simulink library "GainLibrary"  (R2022b)
settings: Solver=VariableStepAuto  StartTime=0.0  StopTime=10.0  RelTol=1e-3
libraries: AudioStats x1
settings Model: Creator=kl13806  LastModifiedBy=kl13806
settings SolverCC: AlgebraicLoopSolver=TrustRegion
settings DebuggingCC: UnconnectedInputMsg=warning  UnconnectedOutputMsg=warning  UnconnectedLineMsg=warning  SFMachineParentedDataDiag=warning  ArithmeticOperatorsInVariantConditions=warning
settings ModelReferenceCC: EnableRefExpFcnMdlSchedulingChecks=on
settings SFSimCC: SimUseLocalCustomCode=off  CustomCodeUndefinedFunction=UseInterfaceOnly
settings RTWCC: RTWUseLocalCustomCode=off  DLArmComputeVersion=19.05
settings CodeAppCC: StateflowObjectComments=on

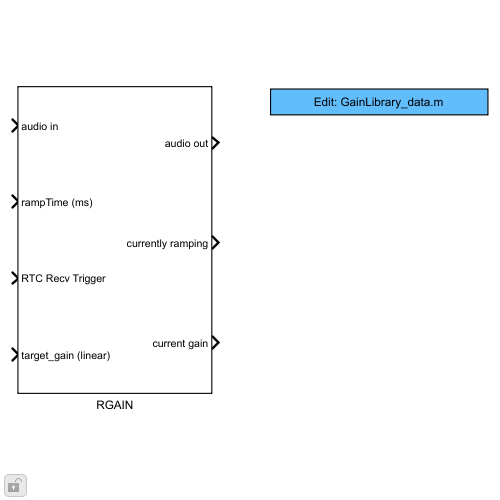
[thumbnail: Simulink's stored preview of the top-level diagram]
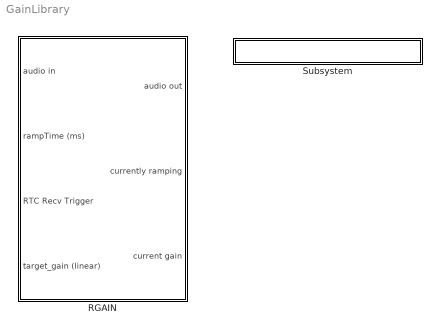
== system GainLibrary ==
  RGAIN : Subsystem  mask(Bose RGAIN){initial_linear_gain=1}
      mask prompts: initial_linear_gain "Initial gain (linear)"
      mask help: The RGAIN block applies a single target gain to all input audio channels.
      mask init:
      | MASK_CONTROL_INIT.frameCount = 0;
      | MASK_CONTROL_INIT.rampCoeff = 1;
      | MASK_CONTROL_INIT.targetGain = initial_linear_gain;
      | MASK_CONTROL_INIT.currentGain = initial_linear_gain;
  Subsystem : Subsystem  mask{filename=GainLibrary_data.m}
      settings: OpenFcn=edit(get(gcbh,'filename'));
      mask Display: disp(['Edit: ' get(gcbh,'filename')]);

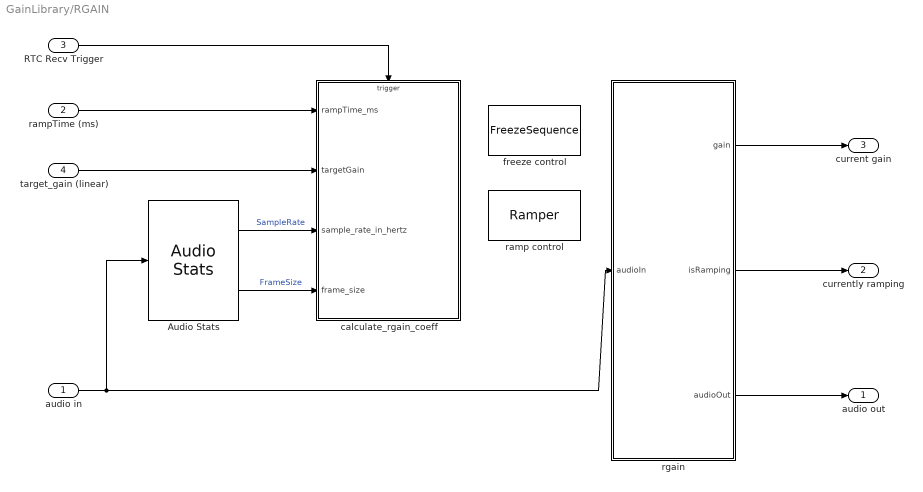
== system GainLibrary/RGAIN ==
  audio in : Inport
  rampTime (ms) : Inport  Port=2
  RTC Recv Trigger : Inport  Port=3
  target_gain (linear) : Inport  Port=4
  Audio Stats : AudioStats/Audio Stats  macroNameRoot=AUDIO  doSampleRate=on  typeSampleRate=Inherit: auto  validateSampleRate=off  valueSampleRate=44100  macroSampleRate=off  doCallRate=off  typeCallRate=Inherit: auto  validateCallRate=off  valueCallRate=[]  macroCallRate=off  doFrameSize=on  typeFrameSize=Inherit: auto  validateFrameSize=off  valueFrameSize=32  macroFrameSize=off  doChannelCount=off  typeChannelCount=Inherit: auto  validateChannelCount=off  valueChannelCount=2  macroChannelCount=off  doTaskRateFactor=off  typeTaskRateFactor=Inherit: auto  validateTaskRateFactor=off  valueTaskRateFactor=[]  macroTaskRateFactor=off  macroTaskID=off
  calculate_rgain_coeff : MATLAB Function  TreatAsAtomicUnit=on
  freeze control : DataStoreMemory  DataStoreName=FreezeSequence  InitialValue=[0,0]  ShowAdditionalParam=off  OutDataTypeStr=uint32
  ramp control : DataStoreMemory  DataStoreName=Ramper  InitialValue=MASK_CONTROL_INIT  ShowAdditionalParam=off  OutDataTypeStr=Bus: rgain_bus
  rgain : MATLAB Function  TreatAsAtomicUnit=on
  audio out : Outport  VectorParamsAs1DForOutWhenUnconnected=off
  currently ramping : Outport  Port=2  VectorParamsAs1DForOutWhenUnconnected=off
  current gain : Outport  Port=3  VectorParamsAs1DForOutWhenUnconnected=off
  wires:
  Audio Stats/1 -> calculate_rgain_coeff/3(sample_rate_in_hertz)  "SampleRate"
  rgain/2(isRamping) -> currently ramping/1
  RTC Recv Trigger/1 -> calculate_rgain_coeff/Trigger
  target_gain (linear)/1 -> calculate_rgain_coeff/2(targetGain)
  rampTime (ms)/1 -> calculate_rgain_coeff/1(rampTime_ms)
  rgain/1(gain) -> current gain/1
  rgain/3(audioOut) -> audio out/1
  audio in/1 -> Audio Stats/1, rgain/1(audioIn)
  Audio Stats/2 -> calculate_rgain_coeff/4(frame_size)  "FrameSize"

== system GainLibrary/Subsystem ==

== matlab function GainLibrary/RGAIN/calculate_rgain_coeff ==
  data: rampTime_ms input; targetGain input; sample_rate_in_hertz input; frame_size input; Ramper data_store_memory; rgain_SILENT_GAIN parameter; FreezeSequence data_store_memory
  events: trigger input FUNCTION_CALL_EVENT
function calculate_rgain_coeff(...
     rampTime_ms, targetGain, sample_rate_in_hertz, frame_size, rgain_SILENT_GAIN)
%#codegen

global Ramper;
global FreezeSequence;


% Step 1: FREEZE the gain ramper so that we can perform calculations based
% on the current gain value. Also, record the control sequence number used
% to specify this soon-to-be-calculated target state.
FreezeSequence(1) = uint32(1); % freeze the gain
FreezeSequence(2) = uint32(1234); % and remember the control sequence (TBD - more changes coming here)

currentGain = Ramper.currentGain;

% Step 2: Nudge the gain values a bit if they are sitting at zero.
% When this control set goes live, ensure that the current gain will move.
% If current gain is zero, replace with a value very close to zero. What we
% really want is a value which is on the edge of perception - not too small
% or large. If the value is too small, we'll waste some of our ramp time
% in perceived silence. If the value is too large, the audio will lurch
% into perceptability at the start of the ramp.
currentGain = max(currentGain, rgain_SILENT_GAIN);

% Step 3: QUANTIZE the desired ramp time to our FrameSize. Also retrieve 
% the whole number of frames required to best match requested ramp time.
% Ensure that at least one frame is used. The frame size will therefore
% determine the steepest ramp (i.e. within one frame you can go anywhere).
quantum_ms = 1000 * frame_size / sample_rate_in_hertz;
numFrames = single(rampTime_ms) / quantum_ms;
numFrames = max (1, round(numFrames));
quantized_rampTime_ms = numFrames * quantum_ms;

%   In order to have the desired ramp time, the slope must vary dependent on the gain difference
%   between target and current value.
%   Ramper's coefficient is therefore calculated as follows:
%                log(TargetGain/CurrentGain)
%   RampCoef = ------------------------------
%                   Fs*(RampTime_ms/1000)
%
factor = log( max(targetGain, rgain_SILENT_GAIN) / currentGain );
RampCoef = exp(factor / (sample_rate_in_hertz * quantized_rampTime_ms / 1000));

% Output asynchronous control signals
Ramper.frameCount   = int32( numFrames );
Ramper.rampCoeff    = single(RampCoef);
Ramper.targetGain   = targetGain;
Ramper.currentGain  = currentGain;

% Release the full rate processing to perform the ramp
FreezeSequence(1) = FreezeSequence(1) - uint32(1);

== matlab function GainLibrary/RGAIN/rgain ==
  data: gain output; isRamping output; audioIn input; audioOut output; Ramper data_store_memory; FreezeSequence data_store_memory
function [gain, isRamping, audioOut]  = rgain(audioIn)
%#codegen

global Ramper;
global FreezeSequence;

% set the size of the output buffer
audioOut = coder.nullcopy(audioIn);

% figure out the frame size
[frame_size, channel_count] = size(audioIn);

% Unpack the control info
frameCount = Ramper.frameCount;
rampCoeff = Ramper.rampCoeff;
targetGain = Ramper.targetGain;
gain = Ramper.currentGain;

% Determine whether gain is ramping or not
% Assume the ramp is frozen
isRamping = false;
k = single(1);

if (FreezeSequence(1) == false)
    if (frameCount == 0)
        % The ramp is finished. Stop ramping and SNAP to the target
        gain = targetGain;
    else
        % The ramp is *NOT* frozen: gain is moving
        isRamping = true;
        k = rampCoeff;
        frameCount = frameCount - 1;
    end
end

for n = 1:frame_size
    gain = gain * k;
    audioOut(n,:) = audioIn(n,:) * gain;
end

% Save state
Ramper.frameCount = frameCount;
Ramper.currentGain = gain;
